simulink model "Finalversion"  (R2019b)
settings: Solver=ode3  StartTime=0.0  StopTime=6009  FixedStep=1  RelTol=1e-3
libraries: sharedutil x3, aerolibconvert2 x2, sharedtransform x2
settings Model: Creator=pieterpinson  LastModifiedBy=pieterpinson
settings DataIOCC: SaveFormat=StructureWithTime
settings OptimizationCC: LifeSpan=inf
settings DebuggingCC: SFExecutionAtInitializationDiag=none  ArithmeticOperatorsInVariantConditions=warning
settings HardwareCC: ProdBitPerSizeT=32  ProdBitPerPtrDiffT=32  ProdWordSize=32  ProdHWDeviceType=Specified
settings SFSimCC: CustomCodeUndefinedFunction=UseInterfaceOnly
settings CodeAppCC: StateflowObjectComments=on

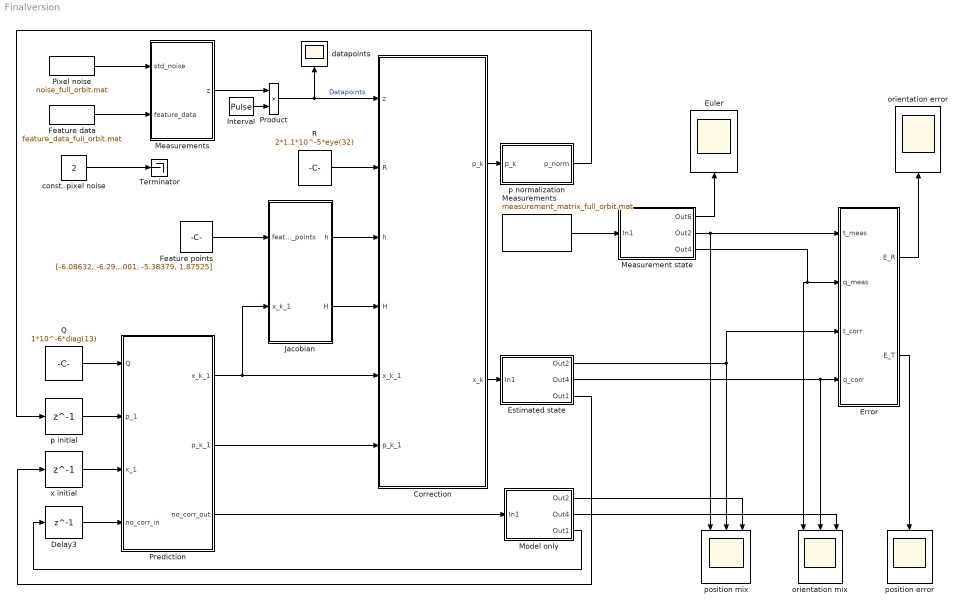
== system Finalversion ==
  " position error" : Scope
  Correction : MATLAB Function  TreatAsAtomicUnit=on
  Delay3 : Delay  DelayLength=1  InitialCondition=[0.208574739540268; 152.898448732150; -0.616785986430221; 0; 0; 0; 0.179685677973094; 0.113609799793228; 0.783094771797942; -0.584438575818727; -0.0873; -0.1489; 0.0262]
  Error : MATLAB Function  TreatAsAtomicUnit=on
  Estimated state : Subsystem
  "Euler " : Scope
  Feature data : FromFile  FileName=feature_data_full_orbit.mat  SampleTime=1
  Feature points : Constant  Value=|
      | [-6.08632, -6.29117, -6.23068, -6.170180, 0.66541, 0.66541, 2.50061, 2.48017, 6.23068, 6.35166, 6.35166, 6.29117,10.84578, 10.82807, 29.52664, 29.55825 ;
      | -0.63573, 1.88967, -0.6022, 1.85389, 2.17147, 2.18343, 3.10581, 3.09464, -0.6368, 2.53604, -0.62563, 2.54752, 2.60307, 1.32946, -8.00742, -9.30518 ;
      | -1.81476, -1.81476, 1.87525, 1.93574, 7.31953, -7.38003, -7.25904, 7.31953, 1.93574, 2.05673, -1.81476, -1.93574, -3.56903, 3.69001, -5.38379, 1.87525]
  Interval : DiscretePulseGenerator  PulseType=Time based  Period=4  PulseWidth=25  PhaseDelay=2
  Jacobian : MATLAB Function  TreatAsAtomicUnit=on
  Measurement state : Subsystem
  Measurements : MATLAB Function  TreatAsAtomicUnit=on
  "Measurements     " : FromFile  FileName=measurement_matrix_full_orbit.mat  SampleTime=1
  Model only : Subsystem
  Pixel noise : FromFile  FileName=noise_full_orbit.mat  SampleTime=1
  Prediction : MATLAB Function  TreatAsAtomicUnit=on
  Product : Product
  Q : Constant  Value=1*10^-6*diag(13)
  R : Constant  Value=2*1.1*10^-5*eye(32)
  Terminator : Terminator
  const. pixel noise : Constant  Value=2
  datapoints : Scope
  orientation mix : Scope  NumInputPorts=3
  orientation error : Scope
  p initial : Delay  DelayLength=1  InitialCondition=|
      | 1*diag([0.210700926920923; 1.80934981153197;
      | 0.618108041852614;
      | 0.0001;
      | 0.0001;
      | 0.0001;
      | 0.0505371300828058;
      | 0.0297889194292068;
      | 0.147292176069403;
      | 0.138188108743277;
      | 0.0001;
      | 0.0001;
      | 0.0001])
  p normalization : MATLAB Function  TreatAsAtomicUnit=on
  position mix : Scope  NumInputPorts=3
  x initial : Delay  DelayLength=1  InitialCondition=[0.208574739540268; 152.898448732150; -0.616785986430221; 0; 0; 0; 0.179685677973094; 0.113609799793228; 0.783094771797942; -0.584438575818727; -0.0873; -0.1489; 0.0262]
  wires:
  Prediction/1(x_k_1) -> Correction/5(x_k_1), Jacobian/2(x_k_1)
  x initial/1 -> Prediction/3(x_1)
  Q/1 -> Prediction/1(Q)
  p initial/1 -> Prediction/2(p_1)
  Prediction/2(p_k_1) -> Correction/6(p_k_1)
  R/1 -> Correction/2(R)
  Feature points/1 -> Jacobian/1(feature_points)
  Delay3/1 -> Prediction/4(no_corr_in)
  Prediction/3(no_corr_out) -> Model only/1(In1)
  Model only/3(Out1) -> Delay3/1
  Correction/2(x_k) -> Estimated state/1(In1)
  Estimated state/3(Out1) -> x initial/1
  Measurement state/2(Out2) -> Error/1(t_meas), position mix/1
  Measurement state/1(Out6) -> "Euler "/1
  Error/2(E_T) -> " position error"/1
  Jacobian/2(H) -> Correction/4(H)
  Estimated state/2(Out4) -> Error/4(q_corr), orientation mix/2
  "Measurements     "/1 -> Measurement state/1(In1)
  Estimated state/1(Out2) -> Error/3(t_corr), position mix/2
  Error/1(E_R) -> orientation error/1
  Correction/1(p_k) -> p normalization/1(p_k)
  Jacobian/1(h) -> Correction/3(h)
  p normalization/1(p_norm) -> p initial/1
  Feature data/1 -> Measurements/2(feature_data)
  Measurement state/3(Out4) -> Error/2(q_meas), orientation mix/1
  Interval/1 -> Product/2
  Measurements/1(z) -> Product/1
  Product/1 -> Correction/1(z), datapoints/1  "Datapoints"
  Pixel noise/1 -> Measurements/1(std_noise)
  Model only/1(Out2) -> position mix/3
  Model only/2(Out4) -> orientation mix/3
  const. pixel noise/1 -> Terminator/1

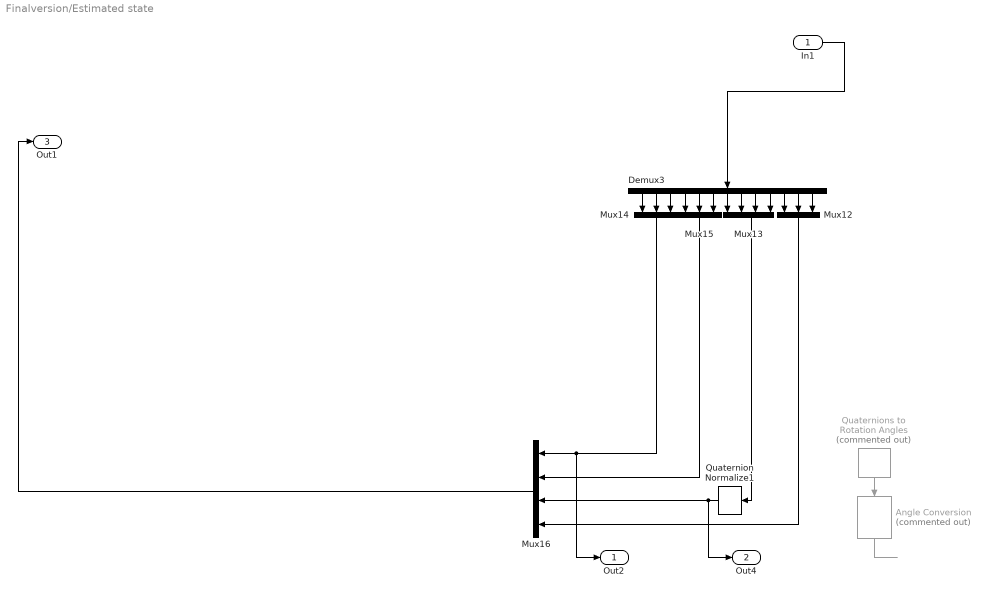
== system Finalversion/Estimated state ==
  In1 : Inport
  Angle Conversion : aerolibconvert2/Angle Conversion  Commented=on  IU=rad  OU=deg
  Demux3 : Demux  Outputs=13
  Mux12 : Mux  Inputs=3
  Mux13 : Mux
  Mux14 : Mux  Inputs=3
  Mux15 : Mux  Inputs=3
  Mux16 : Mux
  Quaternion Normalize1 : sharedutil/Quaternion Normalize  aMode=aMode
      settings: SourceProductName=Aerospace Blockset  SourceProductBaseCode=AE
  Quaternions to Rotation Angles : sharedtransform/Quaternions to Rotation Angles  Commented=on  rotationOrder=ZYX  aMode=aMode
      settings: SourceProductBaseCode=AE
  Out2 : Outport
  Out4 : Outport  Port=2
  Out1 : Outport  Port=3
  wires:
  Mux15/1 -> Mux16/2
  Demux3/2 -> Mux14/2
  Mux14/1 -> Out2/1, Mux16/1
  Quaternion Normalize1/1 -> Out4/1, Mux16/3
  Quaternions to Rotation Angles/1 -> Angle Conversion/1
  In1/1 -> Demux3/1
  Mux13/1 -> Quaternion Normalize1/1
  Demux3/8 -> Mux13/2
  Demux3/1 -> Mux14/1
  Demux3/4 -> Mux15/1
  Mux12/1 -> Mux16/4
  Demux3/7 -> Mux13/1
  Demux3/6 -> Mux15/3
  Demux3/3 -> Mux14/3
  Demux3/5 -> Mux15/2
  Demux3/11 -> Mux12/1
  Demux3/9 -> Mux13/3
  Demux3/10 -> Mux13/4
  Demux3/12 -> Mux12/2
  Demux3/13 -> Mux12/3
  Mux16/1 -> Out1/1
  Angle Conversion/1 -> ?

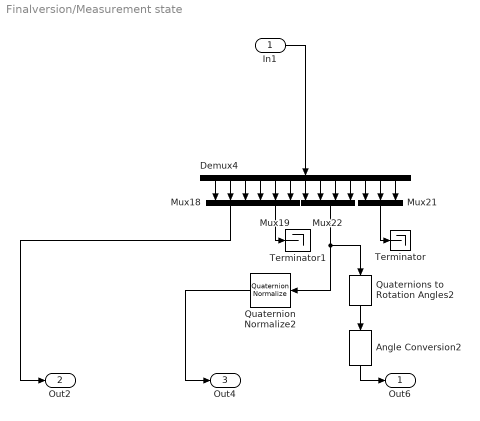
== system Finalversion/Measurement state ==
  In1 : Inport
  Angle Conversion2 : aerolibconvert2/Angle Conversion  IU=rad  OU=deg
  Demux4 : Demux  Outputs=13
  Mux18 : Mux  Inputs=3
  Mux19 : Mux  Inputs=3
  Mux21 : Mux  Inputs=3
  Mux22 : Mux
  Quaternion Normalize2 : sharedutil/Quaternion Normalize  aMode=aMode
      settings: SourceProductName=Aerospace Blockset  SourceProductBaseCode=AE
  Quaternions to Rotation Angles2 : sharedtransform/Quaternions to Rotation Angles  rotationOrder=ZYX  aMode=aMode
      settings: SourceProductBaseCode=AE
  Terminator : Terminator
  Terminator1 : Terminator
  Out6 : Outport
  Out2 : Outport  Port=2
  Out4 : Outport  Port=3
  wires:
  Mux22/1 -> Quaternion Normalize2/1, Quaternions to Rotation Angles2/1
  Demux4/13 -> Mux21/3
  Demux4/8 -> Mux22/2
  Demux4/1 -> Mux18/1
  Quaternion Normalize2/1 -> Out4/1
  Demux4/10 -> Mux22/4
  Demux4/5 -> Mux19/2
  Demux4/11 -> Mux21/1
  Demux4/2 -> Mux18/2
  Demux4/7 -> Mux22/1
  Demux4/12 -> Mux21/2
  Mux18/1 -> Out2/1
  Demux4/3 -> Mux18/3
  Quaternions to Rotation Angles2/1 -> Angle Conversion2/1
  Demux4/9 -> Mux22/3
  Demux4/4 -> Mux19/1
  Demux4/6 -> Mux19/3
  In1/1 -> Demux4/1
  Angle Conversion2/1 -> Out6/1
  Mux19/1 -> Terminator1/1
  Mux21/1 -> Terminator/1

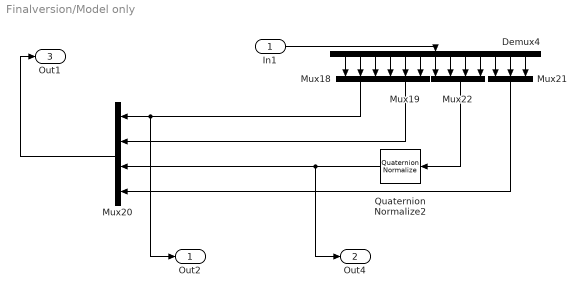
== system Finalversion/Model only ==
  In1 : Inport
  Demux4 : Demux  Outputs=13
  Mux18 : Mux  Inputs=3
  Mux19 : Mux  Inputs=3
  Mux20 : Mux
  Mux21 : Mux  Inputs=3
  Mux22 : Mux
  Quaternion Normalize2 : sharedutil/Quaternion Normalize  aMode=aMode
      settings: SourceProductName=Aerospace Blockset  SourceProductBaseCode=AE
  Out2 : Outport
  Out4 : Outport  Port=2
  Out1 : Outport  Port=3
  wires:
  Mux21/1 -> Mux20/4
  Mux22/1 -> Quaternion Normalize2/1
  Demux4/13 -> Mux21/3
  Demux4/8 -> Mux22/2
  Demux4/1 -> Mux18/1
  Quaternion Normalize2/1 -> Out4/1, Mux20/3
  Mux19/1 -> Mux20/2
  Demux4/10 -> Mux22/4
  Demux4/5 -> Mux19/2
  Demux4/11 -> Mux21/1
  Demux4/2 -> Mux18/2
  Demux4/7 -> Mux22/1
  Demux4/12 -> Mux21/2
  Mux18/1 -> Out2/1, Mux20/1
  Demux4/3 -> Mux18/3
  Demux4/9 -> Mux22/3
  Demux4/4 -> Mux19/1
  Demux4/6 -> Mux19/3
  In1/1 -> Demux4/1
  Mux20/1 -> Out1/1

== matlab function Finalversion/Measurements ==
  data: z output; std_noise input; feature_data input
function z = measurements(std_noise,feature_data)
   
    %import and convert featured data points 
    datapoints = feature_data(:,1);
    z = zeros(32,1);
    
    pixel_size = 1.1*10^-5;
    
    %number of featurepoints
    n = 16;
    
    if std_noise == 0
        for i=1:2*n
        
            z(i,1) = 0;

        end
    else
        for i=1:2*n
        
            z(i,1) = pixel_size*(datapoints(i) + std_noise);

        end
    end
    
end

== matlab function Finalversion/Prediction ==
  data: x_k_1 output; Q input; p_1 input; p_k_1 output; x_1 input; no_corr_in input; no_corr_out output
function [x_k_1,p_k_1,no_corr_out]= prediction(Q,p_1,x_1,no_corr_in)

%orbital parameter
mu = 3.986*10^14;
R_earth = 6371000;
H_target = 773000;
a = R_earth + H_target;
n = sqrt(mu/(a^3));

%clohessy-wiltshire equations
dr = [4-3*cos(n) 0 0 sin(n)/n 2*(1-cos(n))/n 0 ; 6*(sin(n)-n) 1 0 2*(cos(n)-1)/n (4*sin(n)-3*n)/n 0 ; 0 0 cos(n) 0 0 sin(n)/n];
dv = [3*n*sin(n) 0 0 cos(n) 2*sin(n) 0 ; 6*n*(cos(n)-1) 0 0 -2*sin(n) 4*cos(n)-3 0 ; 0 0 -n*sin(n) 0 0 cos(n)];

%quaternion kinematic equation
wq = eul2quat(x_1(11:13)','XYZ'); % This is the unit quaternion rotation due to omega
dq = [wq(1) -wq(2) -wq(3) -wq(4) ; wq(2) wq(1) wq(4) -wq(3) ; wq(3) -wq(4) wq(1) wq(2) ; wq(4) wq(3) -wq(2) wq(1)];

%state transition matrix
fi = [dr zeros(3,7) ; dv zeros(3,7) ; zeros(4,6) dq zeros(4,3) ; zeros(3,10) eye(3)];

%propogation step
x_k_1 = fi * x_1;
p_k_1 = fi * p_1 * fi.' + Q;

%dynamical model only propagation
Phi_wq = [0.9962 ; -0.0445 ; -0.0737 ; 0.0163];
Phi_dq = [Phi_wq(1) -Phi_wq(2) -Phi_wq(3) -Phi_wq(4) ; Phi_wq(2) Phi_wq(1) Phi_wq(4) -Phi_wq(3) ; Phi_wq(3) -Phi_wq(4) Phi_wq(1) Phi_wq(2) ; Phi_wq(4) Phi_wq(3) -Phi_wq(2) Phi_wq(1)];
Phi = [dr zeros(3,7) ; dv zeros(3,7) ; zeros(4,6) Phi_dq zeros(4,3) ; zeros(3,10) eye(3)];
no_corr_out = Phi * no_corr_in;

end

== matlab function Finalversion/Correction ==
  data: z input; R input; h input; p_k output; x_k output; H input; x_k_1 input; p_k_1 input
function [p_k,x_k]= correction(z,R,h,H,x_k_1,p_k_1)

%kalman gain calculation
K = p_k_1 * H' * inv(H * p_k_1 * H' + R);

%correction step
x_k = x_k_1 + K*(z - h);
p_k = (eye(13,13) - K*H)*p_k_1;

end

== matlab function Finalversion/Jacobian ==
  data: feature_points input; h output; x_k_1 input; H output
function [h,H]= Jacobian(feature_points,x_k_1)
    
    %focal length of the camera
    fx = 2*3.9*10^-3;
    fy = 2*3.9*10^-3;
    
    pixel_size = 1.1*10^-5;
    
    %number of featurepoints
    n = 16;

    %individual vector definition
    vectorJacobian = zeros(2*n, 3);
    quaternionJacobian = zeros(2*n, 4);
    h = zeros(32,1);
    
    %import and convert featured data points
    wireframe = feature_points;
    
    for i = 1:n
        
        %quaternion rotation matrix
        q = x_k_1(7:10);
        R_q = quat2rotm(q');
         
        %position vector
        xyz = R_q* wireframe(:,i) + [x_k_1(1); x_k_1(3) ;x_k_1(2)];
        
        %h vector calculation
        h(2*i-1,1) = xyz(1)/xyz(3)*fx + 256*pixel_size;
        h(2*i,1) = xyz(2)/xyz(3)*fy + 256*pixel_size;
        
        %position Jacobian calculation
        vectorJacobian(i*2-1:i*2,1:3) = [fx/xyz(3) 0 -fx*xyz(1)/xyz(3)^2 ; 0 fy/xyz(3) -fy*xyz(2)/xyz(3)^2];
        
        %quaternion rotation Jacobian calculation
        dH_dq_1 = [2*q(1) -2*q(4) 2*q(3); 2*q(4) 2*q(1) -2*q(2); -2*q(3) 2*q(2) 2*q(1)]*xyz;
        dH_dq_2 = [2*q(2) 2*q(3) 2*q(4); 2*q(3) -2*q(2) -2*q(1); 2*q(4) 2*q(1) -2*q(2)]*xyz;
        dH_dq_3 = [-2*q(3) 2*q(2) 2*q(1); 2*q(2) 2*q(3) 2*q(4); -2*q(1) 2*q(4) -2*q(3)]*xyz;
        dH_dq_4 = [-2*q(4) -2*q(1) 2*q(2); 2*q(1) -2*q(4) 2*q(3); 2*q(1) 2*q(3) 2*q(4)]*xyz;
        dH_dq = [dH_dq_1 dH_dq_2 dH_dq_3 dH_dq_4] * [1 0 0 0; 0 -1 0 0; 0 0 -1 0; 0 0 0 -1];
        
        quaternionJacobian(i*2-1:i*2,1:4) = vectorJacobian(i*2-1:i*2,1:3)*dH_dq;
        
    end
    
    %final Jacobian vector
    H = [vectorJacobian, zeros(2*n, 3), quaternionJacobian, zeros(2*n, 3)];

end

== matlab function Finalversion/Error ==
  data: t_meas input; q_meas input; t_corr input; E_R output; q_corr input; E_T output
function [E_R,E_T] = error(t_meas,q_meas,t_corr,q_corr)

    
    Beta = quatmultiply(q_meas', q_corr');
     
    % 
    E_T = abs(t_meas - t_corr);
    E_R = 2*acos(abs(Beta(1)));

end

== matlab function Finalversion/p normalization ==
  data: p_k input; p_norm output
function p_norm = norm(p_k)
    
    %quaternion rotation matrix
    q = [p_k(7,7) ; p_k(8,8) ; p_k(9,9) ; p_k(10,10)];
    q_r = [q(2)^2+q(3)^2+q(4)^2 , -q(1)*q(2), -q(1)*q(3), -q(1)*q(4) ;
        -q(2)*q(1), q(1)^2+q(3)^2+q(4)^2, -q(2)*q(3), -q(2)*q(4) ; 
        -q(3)*q(1), -q(3)*q(2), q(1)^2+q(2)^2+q(4)^2, -q(3)*q(4) ; 
        -q(4)*q(1), -q(4)*q(2), -q(4)*q(3), q(1)^2+q(2)^2+q(3)^2];
    
    %quaternion normalization
    dq_norm = (q(1)^2 + q(2)^2 + q(3)^2 + q(4)^2)^(-3/2) * q_r;
    
    %transformation step
    J = [eye(6) zeros(6,7) ; zeros(4,6) dq_norm zeros(4,3); zeros(3,10) eye(3)];
    p_norm = J * p_k * J';

end
